simulink model "Three_blade_H_VAWT_Model"  (R2018b)
settings: Solver=FixedStepAuto  StartTime=0.0  StopTime=10  FixedStep=0.01  RelTol=1e-3
values from neighbouring files (symbols this model uses):
  A0 = 0    [Three_blade_H_VAWT_init.m]    (also in Three_blade_H_VAWT_pre_post.m)
  a1 = 0.01    [Three_blade_H_VAWT_init.m]    (also in Three_blade_H_VAWT_pre_post.m)
  a11 = 0.8    [Three_blade_H_VAWT_init.m]    (also in Three_blade_H_VAWT_pre_post.m)
  a12 = 0.2    [Three_blade_H_VAWT_init.m]    (also in Three_blade_H_VAWT_pre_post.m)
  a2 = 0.08    [Three_blade_H_VAWT_init.m]    (also in Three_blade_H_VAWT_pre_post.m)
  a21 = 0.5    [Three_blade_H_VAWT_init.m]    (also in Three_blade_H_VAWT_pre_post.m)
  a22 = 0.5    [Three_blade_H_VAWT_init.m]    (also in Three_blade_H_VAWT_pre_post.m)
  A_wind = 10    [Three_blade_H_VAWT_init.m]    (also in Three_blade_H_VAWT_pre_post.m)
  ACD1 = 12    [Three_blade_H_VAWT_init.m]    (also in Three_blade_H_VAWT_pre_post.m)
  ACL1 = 15    [Three_blade_H_VAWT_init.m]    (also in Three_blade_H_VAWT_pre_post.m)
  AR = Blade_Length/Chord    (= 10)    [Three_blade_H_VAWT_init.m]    (also in Three_blade_H_VAWT_pre_post.m = 40)
  blade1_pitch = 0    [Three_blade_H_VAWT_pre_post.m]
  blade1_radius = 20    [Three_blade_H_VAWT_pre_post.m]
  blade2_pitch = 0    [Three_blade_H_VAWT_pre_post.m]
  blade2_radius = 20    [Three_blade_H_VAWT_pre_post.m]
  blade3_pitch = 0    [Three_blade_H_VAWT_pre_post.m]
  blade3_radius = 20    [Three_blade_H_VAWT_pre_post.m]
  Blade_Length = 40    [Three_blade_H_VAWT_init.m]    (also in Three_blade_H_VAWT_pre_post.m)
  C_l_NACA0012_spline = spline(angles, C_l_NACA0012, [0:1:360])    [Three_blade_H_VAWT_init.m]    (also in Three_blade_H_VAWT_pre_post.m)
  CD0 = 0.005    [Three_blade_H_VAWT_init.m]    (also in Three_blade_H_VAWT_pre_post.m)
  CD1_max = 0.017    [Three_blade_H_VAWT_init.m]    (also in Three_blade_H_VAWT_pre_post.m)
  CD2_max = 1.8    [Three_blade_H_VAWT_init.m]    (also in Three_blade_H_VAWT_pre_post.m)
  CL1_max = 1.4    [Three_blade_H_VAWT_init.m]    (also in Three_blade_H_VAWT_pre_post.m)
  CL2_max = 1.2    [Three_blade_H_VAWT_init.m]    (also in Three_blade_H_VAWT_pre_post.m)
  D = 10^6    (= 1000000)    [Three_blade_H_VAWT_init.m]    (also in Three_blade_H_VAWT_pre_post.m)
  eta_g = 0.9    [Three_blade_H_VAWT_init.m]    (also in Three_blade_H_VAWT_pre_post.m)
  h1 = 1    [Three_blade_H_VAWT_init.m]    (also in Three_blade_H_VAWT_pre_post.m)
  h2 = 1    [Three_blade_H_VAWT_init.m]    (also in Three_blade_H_VAWT_pre_post.m)
  Jg = 15.8    [Three_blade_H_VAWT_init.m]    (also in Three_blade_H_VAWT_pre_post.m)
  K = 6*10^7    (= 60000000)    [Three_blade_H_VAWT_init.m]    (also in Three_blade_H_VAWT_pre_post.m)
  N = 100    [Three_blade_H_VAWT_init.m]    (also in Three_blade_H_VAWT_pre_post.m)
  phi11 = 0    [Three_blade_H_VAWT_init.m]    (also in Three_blade_H_VAWT_pre_post.m)
  phi12 = pi/2    (= 1.57079632679)    [Three_blade_H_VAWT_init.m]    (also in Three_blade_H_VAWT_pre_post.m)
  phi21 = 0    [Three_blade_H_VAWT_init.m]    (also in Three_blade_H_VAWT_pre_post.m)
  phi22 = pi/2    (= 1.57079632679)    [Three_blade_H_VAWT_init.m]    (also in Three_blade_H_VAWT_pre_post.m)
  Planform_A = Blade_Length*Chord    (= 160)    [Three_blade_H_VAWT_init.m]    (also in Three_blade_H_VAWT_pre_post.m = 40)
  rho = 1.225    [Three_blade_H_VAWT_init.m]    (also in Three_blade_H_VAWT_pre_post.m; sim_init_junior_project.m)
  S1 = 0.6/6    (= 0.1)    [Three_blade_H_VAWT_init.m]    (also in Three_blade_H_VAWT_pre_post.m)
  v_gustmax = v_wind    (= 5)    [Three_blade_H_VAWT_init.m]    (also in Three_blade_H_VAWT_pre_post.m)
  v_wind = 5    [Three_blade_H_VAWT_init.m]    (also in Three_blade_H_VAWT_pre_post.m)
  w_gust = (2*pi)/(30)    (= 0.209439510239)    [Three_blade_H_VAWT_init.m]    (also in Three_blade_H_VAWT_pre_post.m)
  w_wind = (2*pi)*5    (= 31.4159265359)    [Three_blade_H_VAWT_init.m]    (also in Three_blade_H_VAWT_pre_post.m)
  wind_vector_i = [50,0,0]    [Three_blade_H_VAWT_pre_post.m]
undefined symbols (not defined in the file or in its folder): Bg, C_Tg, C_Tr, c_wg, c_wr, Cg, Cr, J_g, Kg, Kr, L, magnitude, R2, Re, tau_e
libraries: vrlib x6, dspmathops x6
(part 2 of 2)

== system Three_blade_H_VAWT_Model/3bladeHVAWT with Generator/Blade Aerodymanics/Pre//Post Stall Foil Model NACA 0012/CD2 (post-stall) 1 ==
  alpha : Inport
  Abs : Abs
  CD2_max : Constant  Value=CD2_max
  Constant : Constant  Value=CD1_max
  Constant1 : Constant  Value=ACD1
  Constant2 : Constant  Value=90
  Constant3 : Constant  Value=ACD1
  Divide : Product  Inputs=**/
  Gain : Gain  Gain=pi/180
  MATLAB Function : MATLAB Function  TreatAsAtomicUnit=on
  Product : Product
  Product1 : Product
  Scope : Scope
  Sum : Sum  Inputs=|++
  Sum1 : Sum  Inputs=|+-
  Sum2 : Sum  Inputs=|+-
  Sum3 : Sum  Inputs=|+-
  Trigonometric Function : Trigonometry
  Cd : Outport
  wires:
  Constant/1 -> Sum/2, Sum1/2
  CD2_max/1 -> Sum1/1
  Sum1/1 -> Product/2
  Trigonometric Function/1 -> Product/1
  Product/1 -> Sum/1
  alpha/1 -> MATLAB Function/1(alpha), Sum2/1
  Constant1/1 -> Sum3/2, Sum2/2
  Constant2/1 -> Divide/2, Sum3/1
  Sum3/1 -> Divide/3
  Sum2/1 -> Divide/1
  Divide/1 -> Gain/1
  Gain/1 -> Trigonometric Function/1
  Product1/1 -> Abs/1
  Abs/1 -> Cd/1
  Constant3/1 -> MATLAB Function/2(ACD1)
  Sum/1 -> Product1/2
  MATLAB Function/1(y) -> Scope/1, Product1/1

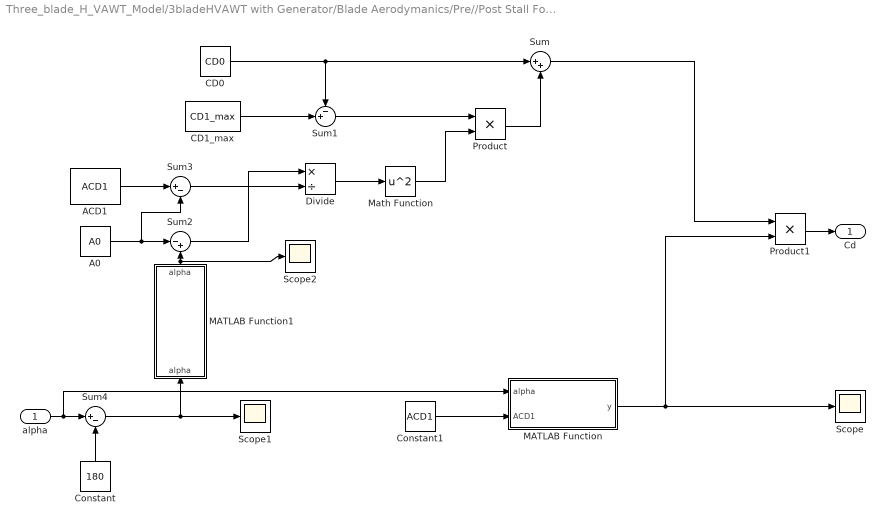
== system Three_blade_H_VAWT_Model/3bladeHVAWT with Generator/Blade Aerodymanics/Pre//Post Stall Foil Model NACA 0012/CD2 (post-stall) 2 ==
  alpha : Inport
  A0 : Constant  Value=A0
  ACD1 : Constant  Value=ACD1
  CD0 : Constant  Value=CD0
  CD1_max : Constant  Value=CD1_max
  Constant : Constant  Value=180
  Constant1 : Constant  Value=ACD1
  Divide : Product  Inputs=*/
  MATLAB Function : MATLAB Function  TreatAsAtomicUnit=on
  MATLAB Function1 : MATLAB Function  TreatAsAtomicUnit=on
  Math Function : Math  Operator=square  SaturateOnIntegerOverflow=on
  Product : Product
  Product1 : Product
  Scope : Scope
  Scope1 : Scope
  Scope2 : Scope
  Sum : Sum  Inputs=|++
  Sum1 : Sum  Inputs=-+|
  Sum2 : Sum  Inputs=|-+
  Sum3 : Sum  Inputs=|+-
  Sum4 : Sum  Inputs=|+-
  Cd : Outport
  wires:
  MATLAB Function1/1(alpha) -> Sum2/2, Scope2/1
  MATLAB Function/1(y) -> Scope/1, Product1/2
  Constant1/1 -> MATLAB Function/2(ACD1)
  Product1/1 -> Cd/1
  Sum/1 -> Product1/1
  Product/1 -> Sum/2
  Math Function/1 -> Product/2
  Divide/1 -> Math Function/1
  Sum3/1 -> Divide/2
  Sum2/1 -> Divide/1
  ACD1/1 -> Sum3/1
  A0/1 -> Sum2/1, Sum3/2
  Sum1/1 -> Product/1
  CD1_max/1 -> Sum1/2
  CD0/1 -> Sum/1, Sum1/1
  alpha/1 -> MATLAB Function/1(alpha), Sum4/1
  Sum4/1 -> Scope1/1, MATLAB Function1/1("alpha ")
  Constant/1 -> Sum4/2

== system Three_blade_H_VAWT_Model/3bladeHVAWT with Generator/Blade Aerodymanics/Pre//Post Stall Foil Model NACA 0012/CD2 (post-stall) 3 ==
  alpha : Inport
  Abs : Abs
  CD2_max : Constant  Value=CD2_max
  Constant : Constant  Value=CD1_max
  Constant1 : Constant  Value=ACD1
  Constant2 : Constant  Value=90
  Constant3 : Constant  Value=ACD1
  Constant4 : Constant  Value=-180
  Divide : Product  Inputs=**/
  Gain : Gain  Gain=pi/180
  MATLAB Function : MATLAB Function  TreatAsAtomicUnit=on
  Product : Product
  Product1 : Product
  Scope : Scope
  Sum : Sum  Inputs=|++
  Sum1 : Sum  Inputs=|+-
  Sum2 : Sum  Inputs=|+-
  Sum3 : Sum  Inputs=|+-
  Sum4 : Sum  Inputs=++|
  Trigonometric Function : Trigonometry
  Cd : Outport
  wires:
  MATLAB Function/1(y) -> Product1/1, Scope/1
  Sum/1 -> Product1/2
  Constant3/1 -> MATLAB Function/2(ACD1)
  Abs/1 -> Cd/1
  Product1/1 -> Abs/1
  Gain/1 -> Trigonometric Function/1
  Divide/1 -> Gain/1
  Sum2/1 -> Sum4/2
  Sum3/1 -> Divide/3
  Constant2/1 -> Sum3/1, Divide/2
  Constant1/1 -> Sum2/2, Sum3/2
  alpha/1 -> Sum2/1, MATLAB Function/1(alpha)
  Product/1 -> Sum/1
  Trigonometric Function/1 -> Product/1
  Sum1/1 -> Product/2
  CD2_max/1 -> Sum1/1
  Constant/1 -> Sum1/2, Sum/2
  Constant4/1 -> Sum4/1
  Sum4/1 -> Divide/1

== system Three_blade_H_VAWT_Model/3bladeHVAWT with Generator/Blade Aerodymanics/Pre//Post Stall Foil Model NACA 0012/CL1 (pre-stall) 1 ==
  alpha : Inport
  A0 : Constant  Value=A0
  A0 1 : Constant  Value=A0
  A0 2 : Constant  Value=A0
  ACl1 : Constant  Value=ACL1
  Cl1max : Constant  Value=CL1_max
  Constant : Constant
  Divide : Product  Inputs=/*
  Divide1 : Product  Inputs=*/
  Math Function : Math  Operator=pow  SaturateOnIntegerOverflow=on
  Product : Product
  Product1 : Product
  Product2 : Product
  S1 : Constant  Value=S1
  Sum{,1,3..4} (4 alike) : Sum  Inputs=|+-
  Sum2 : Sum  Inputs=|++
  Sum5 : Sum  Inputs=-+|
  Cl : Outport
  wires:
  alpha/1 -> Sum3/1
  ACl1/1 -> Sum/1, Sum4/1
  A0/1 -> Sum/2
  Cl1max/1 -> Sum1/2, Divide/2
  Sum/1 -> Product/2
  S1/1 -> Product/1, Product1/2
  Product/1 -> Sum1/1
  Sum1/1 -> Divide/1, Product2/2  "RCl1"
  Divide/1 -> Sum2/1
  Constant/1 -> Sum2/2
  Sum2/1 -> Math Function/2  "N1"
  A0 1/1 -> Sum3/2
  Sum3/1 -> Divide1/1, Product1/1
  Product1/1 -> Sum5/2
  Sum4/1 -> Divide1/2
  A0 2/1 -> Sum4/2
  Divide1/1 -> Math Function/1
  Math Function/1 -> Product2/1
  Product2/1 -> Sum5/1
  Sum5/1 -> Cl/1

== system Three_blade_H_VAWT_Model/3bladeHVAWT with Generator/Blade Aerodymanics/Pre//Post Stall Foil Model NACA 0012/CL2 (post-stall) 1 ==
  alpha : Inport
  Constant : Constant  Value=92
  Constant1 : Constant  Value=1.632
  Constant2 : Constant  Value=CL2_max
  Constant3 : Constant
  Divide : Product  Inputs=*/
  Gain : Gain  Gain=-0.032
  Gain1 : Gain  Gain=-1
  Gain2 : Gain  Gain=-1/51
  Math Function : Math  Operator=pow  SaturateOnIntegerOverflow=on
  Product : Product
  Sum : Sum  Inputs=|+-
  Sum1 : Sum  Inputs=|+-
  Sum2 : Sum  Inputs=|++
  Sum3 : Sum  Inputs=|++
  CL2 : Outport
  wires:
  alpha/1 -> Sum/1
  Constant/1 -> Sum/2
  Sum/1 -> Gain2/1, Gain/1
  Constant1/1 -> Sum1/1
  Constant2/1 -> Sum1/2, Divide/2
  Sum1/1 -> Gain1/1, Divide/1  "RCL2"
  Constant3/1 -> Sum2/1
  Divide/1 -> Sum2/2
  Sum2/1 -> Math Function/2  "N2"
  Gain1/1 -> Product/1
  Gain2/1 -> Math Function/1
  Math Function/1 -> Product/2
  Gain/1 -> Sum3/1
  Product/1 -> Sum3/2
  Sum3/1 -> CL2/1

== system Three_blade_H_VAWT_Model/3bladeHVAWT with Generator/Blade Aerodymanics/Pre//Post Stall Foil Model NACA 0012 (2)/CD1 (pre-stall) 1 ==
  alpha : Inport
  A0 : Constant  Value=A0
  ACD1 : Constant  Value=ACD1
  CD0 : Constant  Value=CD0
  CD1_max : Constant  Value=CD1_max
  Constant1 : Constant  Value=ACD1
  Divide : Product  Inputs=*/
  MATLAB Function : MATLAB Function  TreatAsAtomicUnit=on
  MATLAB Function1 : MATLAB Function  TreatAsAtomicUnit=on
  Math Function : Math  Operator=square  SaturateOnIntegerOverflow=on
  Product : Product
  Product1 : Product
  Scope : Scope
  Scope1 : Scope
  Scope2 : Scope
  Sum : Sum  Inputs=|++
  Sum1 : Sum  Inputs=-+|
  Sum2 : Sum  Inputs=|-+
  Sum3 : Sum  Inputs=|+-
  Cd : Outport
  wires:
  MATLAB Function1/1(alpha) -> Sum2/2, Scope2/1
  MATLAB Function/1(y) -> Scope/1, Product1/2
  Constant1/1 -> MATLAB Function/2(ACD1)
  Product1/1 -> Cd/1
  Sum/1 -> Product1/1
  Product/1 -> Sum/2
  Math Function/1 -> Product/2
  Divide/1 -> Math Function/1
  Sum3/1 -> Divide/2
  Sum2/1 -> Divide/1
  ACD1/1 -> Sum3/1
  A0/1 -> Sum2/1, Sum3/2
  Sum1/1 -> Product/1
  CD1_max/1 -> Sum1/2
  CD0/1 -> Sum/1, Sum1/1
  alpha/1 -> MATLAB Function1/1("alpha "), Scope1/1, MATLAB Function/1(alpha)

== system Three_blade_H_VAWT_Model/3bladeHVAWT with Generator/Blade Aerodymanics/Pre//Post Stall Foil Model NACA 0012 (2)/CD2 (post-stall) 1 ==
  alpha : Inport
  Abs : Abs
  CD2_max : Constant  Value=CD2_max
  Constant : Constant  Value=CD1_max
  Constant1 : Constant  Value=ACD1
  Constant2 : Constant  Value=90
  Constant3 : Constant  Value=ACD1
  Divide : Product  Inputs=**/
  Gain : Gain  Gain=pi/180
  MATLAB Function : MATLAB Function  TreatAsAtomicUnit=on
  Product : Product
  Product1 : Product
  Scope : Scope
  Sum : Sum  Inputs=|++
  Sum1 : Sum  Inputs=|+-
  Sum2 : Sum  Inputs=|+-
  Sum3 : Sum  Inputs=|+-
  Trigonometric Function : Trigonometry
  Cd : Outport
  wires:
  MATLAB Function/1(y) -> Product1/1, Scope/1
  Sum/1 -> Product1/2
  Constant3/1 -> MATLAB Function/2(ACD1)
  Abs/1 -> Cd/1
  Product1/1 -> Abs/1
  Gain/1 -> Trigonometric Function/1
  Divide/1 -> Gain/1
  Sum2/1 -> Divide/1
  Sum3/1 -> Divide/3
  Constant2/1 -> Sum3/1, Divide/2
  Constant1/1 -> Sum2/2, Sum3/2
  alpha/1 -> Sum2/1, MATLAB Function/1(alpha)
  Product/1 -> Sum/1
  Trigonometric Function/1 -> Product/1
  Sum1/1 -> Product/2
  CD2_max/1 -> Sum1/1
  Constant/1 -> Sum1/2, Sum/2

== system Three_blade_H_VAWT_Model/3bladeHVAWT with Generator/Blade Aerodymanics/Pre//Post Stall Foil Model NACA 0012 (2)/CD2 (post-stall) 2 ==
  alpha : Inport
  A0 : Constant  Value=A0
  ACD1 : Constant  Value=ACD1
  CD0 : Constant  Value=CD0
  CD1_max : Constant  Value=CD1_max
  Constant : Constant  Value=180
  Constant1 : Constant  Value=ACD1
  Divide : Product  Inputs=*/
  MATLAB Function : MATLAB Function  TreatAsAtomicUnit=on
  MATLAB Function1 : MATLAB Function  TreatAsAtomicUnit=on
  Math Function : Math  Operator=square  SaturateOnIntegerOverflow=on
  Product : Product
  Product1 : Product
  Scope : Scope
  Scope1 : Scope
  Scope2 : Scope
  Sum : Sum  Inputs=|++
  Sum1 : Sum  Inputs=-+|
  Sum2 : Sum  Inputs=|-+
  Sum3 : Sum  Inputs=|+-
  Sum4 : Sum  Inputs=|+-
  Cd : Outport
  wires:
  Constant/1 -> Sum4/2
  Sum4/1 -> MATLAB Function1/1("alpha "), Scope1/1
  alpha/1 -> Sum4/1, MATLAB Function/1(alpha)
  CD0/1 -> Sum1/1, Sum/1
  CD1_max/1 -> Sum1/2
  Sum1/1 -> Product/1
  A0/1 -> Sum3/2, Sum2/1
  ACD1/1 -> Sum3/1
  Sum2/1 -> Divide/1
  Sum3/1 -> Divide/2
  Divide/1 -> Math Function/1
  Math Function/1 -> Product/2
  Product/1 -> Sum/2
  Sum/1 -> Product1/1
  Product1/1 -> Cd/1
  Constant1/1 -> MATLAB Function/2(ACD1)
  MATLAB Function/1(y) -> Product1/2, Scope/1
  MATLAB Function1/1(alpha) -> Scope2/1, Sum2/2

== system Three_blade_H_VAWT_Model/3bladeHVAWT with Generator/Blade Aerodymanics/Pre//Post Stall Foil Model NACA 0012 (2)/CD2 (post-stall) 3 ==
  alpha : Inport
  Abs : Abs
  CD2_max : Constant  Value=CD2_max
  Constant : Constant  Value=CD1_max
  Constant1 : Constant  Value=ACD1
  Constant2 : Constant  Value=90
  Constant3 : Constant  Value=ACD1
  Constant4 : Constant  Value=-180
  Divide : Product  Inputs=**/
  Gain : Gain  Gain=pi/180
  MATLAB Function : MATLAB Function  TreatAsAtomicUnit=on
  Product : Product
  Product1 : Product
  Scope : Scope
  Sum : Sum  Inputs=|++
  Sum1 : Sum  Inputs=|+-
  Sum2 : Sum  Inputs=|+-
  Sum3 : Sum  Inputs=|+-
  Sum4 : Sum  Inputs=++|
  Trigonometric Function : Trigonometry
  Cd : Outport
  wires:
  Sum4/1 -> Divide/1
  Constant4/1 -> Sum4/1
  Constant/1 -> Sum/2, Sum1/2
  CD2_max/1 -> Sum1/1
  Sum1/1 -> Product/2
  Trigonometric Function/1 -> Product/1
  Product/1 -> Sum/1
  alpha/1 -> MATLAB Function/1(alpha), Sum2/1
  Constant1/1 -> Sum3/2, Sum2/2
  Constant2/1 -> Divide/2, Sum3/1
  Sum3/1 -> Divide/3
  Sum2/1 -> Sum4/2
  Divide/1 -> Gain/1
  Gain/1 -> Trigonometric Function/1
  Product1/1 -> Abs/1
  Abs/1 -> Cd/1
  Constant3/1 -> MATLAB Function/2(ACD1)
  Sum/1 -> Product1/2
  MATLAB Function/1(y) -> Scope/1, Product1/1

== system Three_blade_H_VAWT_Model/3bladeHVAWT with Generator/Blade Aerodymanics/Pre//Post Stall Foil Model NACA 0012 (2)/CL1 (pre-stall) 1 ==
  alpha : Inport
  A0 : Constant  Value=A0
  A0 1 : Constant  Value=A0
  A0 2 : Constant  Value=A0
  ACl1 : Constant  Value=ACL1
  Cl1max : Constant  Value=CL1_max
  Constant : Constant
  Divide : Product  Inputs=/*
  Divide1 : Product  Inputs=*/
  Math Function : Math  Operator=pow  SaturateOnIntegerOverflow=on
  Product : Product
  Product1 : Product
  Product2 : Product
  S1 : Constant  Value=S1
  Sum{,1,3..4} (4 alike) : Sum  Inputs=|+-
  Sum2 : Sum  Inputs=|++
  Sum5 : Sum  Inputs=-+|
  Cl : Outport
  wires:
  Sum5/1 -> Cl/1
  Product2/1 -> Sum5/1
  Math Function/1 -> Product2/1
  Divide1/1 -> Math Function/1
  A0 2/1 -> Sum4/2
  Sum4/1 -> Divide1/2
  Product1/1 -> Sum5/2
  Sum3/1 -> Product1/1, Divide1/1
  A0 1/1 -> Sum3/2
  Sum2/1 -> Math Function/2  "N1"
  Constant/1 -> Sum2/2
  Divide/1 -> Sum2/1
  Sum1/1 -> Product2/2, Divide/1  "RCl1"
  Product/1 -> Sum1/1
  S1/1 -> Product1/2, Product/1
  Sum/1 -> Product/2
  Cl1max/1 -> Divide/2, Sum1/2
  A0/1 -> Sum/2
  ACl1/1 -> Sum4/1, Sum/1
  alpha/1 -> Sum3/1

== system Three_blade_H_VAWT_Model/3bladeHVAWT with Generator/Blade Aerodymanics/Pre//Post Stall Foil Model NACA 0012 (2)/CL2 (post-stall) 1 ==
  alpha : Inport
  Constant : Constant  Value=92
  Constant1 : Constant  Value=1.632
  Constant2 : Constant  Value=CL2_max
  Constant3 : Constant
  Divide : Product  Inputs=*/
  Gain : Gain  Gain=-0.032
  Gain1 : Gain  Gain=-1
  Gain2 : Gain  Gain=-1/51
  Math Function : Math  Operator=pow  SaturateOnIntegerOverflow=on
  Product : Product
  Sum : Sum  Inputs=|+-
  Sum1 : Sum  Inputs=|+-
  Sum2 : Sum  Inputs=|++
  Sum3 : Sum  Inputs=|++
  CL2 : Outport
  wires:
  Sum3/1 -> CL2/1
  Product/1 -> Sum3/2
  Gain/1 -> Sum3/1
  Math Function/1 -> Product/2
  Gain2/1 -> Math Function/1
  Gain1/1 -> Product/1
  Sum2/1 -> Math Function/2  "N2"
  Divide/1 -> Sum2/2
  Constant3/1 -> Sum2/1
  Sum1/1 -> Divide/1, Gain1/1  "RCL2"
  Constant2/1 -> Divide/2, Sum1/2
  Constant1/1 -> Sum1/1
  Sum/1 -> Gain/1, Gain2/1
  Constant/1 -> Sum/2
  alpha/1 -> Sum/1

== system Three_blade_H_VAWT_Model/3bladeHVAWT with Generator/Blade Aerodymanics/Pre//Post Stall Foil Model NACA 0012 (3)/CD1 (pre-stall) 1 ==
  alpha : Inport
  A0 : Constant  Value=A0
  ACD1 : Constant  Value=ACD1
  CD0 : Constant  Value=CD0
  CD1_max : Constant  Value=CD1_max
  Constant1 : Constant  Value=ACD1
  Divide : Product  Inputs=*/
  MATLAB Function : MATLAB Function  TreatAsAtomicUnit=on
  MATLAB Function1 : MATLAB Function  TreatAsAtomicUnit=on
  Math Function : Math  Operator=square  SaturateOnIntegerOverflow=on
  Product : Product
  Product1 : Product
  Scope : Scope
  Scope1 : Scope
  Scope2 : Scope
  Sum : Sum  Inputs=|++
  Sum1 : Sum  Inputs=-+|
  Sum2 : Sum  Inputs=|-+
  Sum3 : Sum  Inputs=|+-
  Cd : Outport
  wires:
  alpha/1 -> MATLAB Function/1(alpha), Scope1/1, MATLAB Function1/1("alpha ")
  CD0/1 -> Sum1/1, Sum/1
  CD1_max/1 -> Sum1/2
  Sum1/1 -> Product/1
  A0/1 -> Sum3/2, Sum2/1
  ACD1/1 -> Sum3/1
  Sum2/1 -> Divide/1
  Sum3/1 -> Divide/2
  Divide/1 -> Math Function/1
  Math Function/1 -> Product/2
  Product/1 -> Sum/2
  Sum/1 -> Product1/1
  Product1/1 -> Cd/1
  Constant1/1 -> MATLAB Function/2(ACD1)
  MATLAB Function/1(y) -> Product1/2, Scope/1
  MATLAB Function1/1(alpha) -> Scope2/1, Sum2/2

== system Three_blade_H_VAWT_Model/3bladeHVAWT with Generator/Blade Aerodymanics/Pre//Post Stall Foil Model NACA 0012 (3)/CD2 (post-stall) 1 ==
  alpha : Inport
  Abs : Abs
  CD2_max : Constant  Value=CD2_max
  Constant : Constant  Value=CD1_max
  Constant1 : Constant  Value=ACD1
  Constant2 : Constant  Value=90
  Constant3 : Constant  Value=ACD1
  Divide : Product  Inputs=**/
  Gain : Gain  Gain=pi/180
  MATLAB Function : MATLAB Function  TreatAsAtomicUnit=on
  Product : Product
  Product1 : Product
  Scope : Scope
  Sum : Sum  Inputs=|++
  Sum1 : Sum  Inputs=|+-
  Sum2 : Sum  Inputs=|+-
  Sum3 : Sum  Inputs=|+-
  Trigonometric Function : Trigonometry
  Cd : Outport
  wires:
  Constant/1 -> Sum/2, Sum1/2
  CD2_max/1 -> Sum1/1
  Sum1/1 -> Product/2
  Trigonometric Function/1 -> Product/1
  Product/1 -> Sum/1
  alpha/1 -> MATLAB Function/1(alpha), Sum2/1
  Constant1/1 -> Sum3/2, Sum2/2
  Constant2/1 -> Divide/2, Sum3/1
  Sum3/1 -> Divide/3
  Sum2/1 -> Divide/1
  Divide/1 -> Gain/1
  Gain/1 -> Trigonometric Function/1
  Product1/1 -> Abs/1
  Abs/1 -> Cd/1
  Constant3/1 -> MATLAB Function/2(ACD1)
  Sum/1 -> Product1/2
  MATLAB Function/1(y) -> Scope/1, Product1/1

== system Three_blade_H_VAWT_Model/3bladeHVAWT with Generator/Blade Aerodymanics/Pre//Post Stall Foil Model NACA 0012 (3)/CD2 (post-stall) 2 ==
  alpha : Inport
  A0 : Constant  Value=A0
  ACD1 : Constant  Value=ACD1
  CD0 : Constant  Value=CD0
  CD1_max : Constant  Value=CD1_max
  Constant : Constant  Value=180
  Constant1 : Constant  Value=ACD1
  Divide : Product  Inputs=*/
  MATLAB Function : MATLAB Function  TreatAsAtomicUnit=on
  MATLAB Function1 : MATLAB Function  TreatAsAtomicUnit=on
  Math Function : Math  Operator=square  SaturateOnIntegerOverflow=on
  Product : Product
  Product1 : Product
  Scope : Scope
  Scope1 : Scope
  Scope2 : Scope
  Sum : Sum  Inputs=|++
  Sum1 : Sum  Inputs=-+|
  Sum2 : Sum  Inputs=|-+
  Sum3 : Sum  Inputs=|+-
  Sum4 : Sum  Inputs=|+-
  Cd : Outport
  wires:
  MATLAB Function1/1(alpha) -> Sum2/2, Scope2/1
  MATLAB Function/1(y) -> Scope/1, Product1/2
  Constant1/1 -> MATLAB Function/2(ACD1)
  Product1/1 -> Cd/1
  Sum/1 -> Product1/1
  Product/1 -> Sum/2
  Math Function/1 -> Product/2
  Divide/1 -> Math Function/1
  Sum3/1 -> Divide/2
  Sum2/1 -> Divide/1
  ACD1/1 -> Sum3/1
  A0/1 -> Sum2/1, Sum3/2
  Sum1/1 -> Product/1
  CD1_max/1 -> Sum1/2
  CD0/1 -> Sum/1, Sum1/1
  alpha/1 -> MATLAB Function/1(alpha), Sum4/1
  Sum4/1 -> Scope1/1, MATLAB Function1/1("alpha ")
  Constant/1 -> Sum4/2

== system Three_blade_H_VAWT_Model/3bladeHVAWT with Generator/Blade Aerodymanics/Pre//Post Stall Foil Model NACA 0012 (3)/CD2 (post-stall) 3 ==
  alpha : Inport
  Abs : Abs
  CD2_max : Constant  Value=CD2_max
  Constant : Constant  Value=CD1_max
  Constant1 : Constant  Value=ACD1
  Constant2 : Constant  Value=90
  Constant3 : Constant  Value=ACD1
  Constant4 : Constant  Value=-180
  Divide : Product  Inputs=**/
  Gain : Gain  Gain=pi/180
  MATLAB Function : MATLAB Function  TreatAsAtomicUnit=on
  Product : Product
  Product1 : Product
  Scope : Scope
  Sum : Sum  Inputs=|++
  Sum1 : Sum  Inputs=|+-
  Sum2 : Sum  Inputs=|+-
  Sum3 : Sum  Inputs=|+-
  Sum4 : Sum  Inputs=++|
  Trigonometric Function : Trigonometry
  Cd : Outport
  wires:
  MATLAB Function/1(y) -> Product1/1, Scope/1
  Sum/1 -> Product1/2
  Constant3/1 -> MATLAB Function/2(ACD1)
  Abs/1 -> Cd/1
  Product1/1 -> Abs/1
  Gain/1 -> Trigonometric Function/1
  Divide/1 -> Gain/1
  Sum2/1 -> Sum4/2
  Sum3/1 -> Divide/3
  Constant2/1 -> Sum3/1, Divide/2
  Constant1/1 -> Sum2/2, Sum3/2
  alpha/1 -> Sum2/1, MATLAB Function/1(alpha)
  Product/1 -> Sum/1
  Trigonometric Function/1 -> Product/1
  Sum1/1 -> Product/2
  CD2_max/1 -> Sum1/1
  Constant/1 -> Sum1/2, Sum/2
  Constant4/1 -> Sum4/1
  Sum4/1 -> Divide/1

== system Three_blade_H_VAWT_Model/3bladeHVAWT with Generator/Blade Aerodymanics/Pre//Post Stall Foil Model NACA 0012 (3)/CL1 (pre-stall) 1 ==
  alpha : Inport
  A0 : Constant  Value=A0
  A0 1 : Constant  Value=A0
  A0 2 : Constant  Value=A0
  ACl1 : Constant  Value=ACL1
  Cl1max : Constant  Value=CL1_max
  Constant : Constant
  Divide : Product  Inputs=/*
  Divide1 : Product  Inputs=*/
  Math Function : Math  Operator=pow  SaturateOnIntegerOverflow=on
  Product : Product
  Product1 : Product
  Product2 : Product
  S1 : Constant  Value=S1
  Sum{,1,3..4} (4 alike) : Sum  Inputs=|+-
  Sum2 : Sum  Inputs=|++
  Sum5 : Sum  Inputs=-+|
  Cl : Outport
  wires:
  alpha/1 -> Sum3/1
  ACl1/1 -> Sum/1, Sum4/1
  A0/1 -> Sum/2
  Cl1max/1 -> Sum1/2, Divide/2
  Sum/1 -> Product/2
  S1/1 -> Product/1, Product1/2
  Product/1 -> Sum1/1
  Sum1/1 -> Divide/1, Product2/2  "RCl1"
  Divide/1 -> Sum2/1
  Constant/1 -> Sum2/2
  Sum2/1 -> Math Function/2  "N1"
  A0 1/1 -> Sum3/2
  Sum3/1 -> Divide1/1, Product1/1
  Product1/1 -> Sum5/2
  Sum4/1 -> Divide1/2
  A0 2/1 -> Sum4/2
  Divide1/1 -> Math Function/1
  Math Function/1 -> Product2/1
  Product2/1 -> Sum5/1
  Sum5/1 -> Cl/1

== system Three_blade_H_VAWT_Model/3bladeHVAWT with Generator/Blade Aerodymanics/Pre//Post Stall Foil Model NACA 0012 (3)/CL2 (post-stall) 1 ==
  alpha : Inport
  Constant : Constant  Value=92
  Constant1 : Constant  Value=1.632
  Constant2 : Constant  Value=CL2_max
  Constant3 : Constant
  Divide : Product  Inputs=*/
  Gain : Gain  Gain=-0.032
  Gain1 : Gain  Gain=-1
  Gain2 : Gain  Gain=-1/51
  Math Function : Math  Operator=pow  SaturateOnIntegerOverflow=on
  Product : Product
  Sum : Sum  Inputs=|+-
  Sum1 : Sum  Inputs=|+-
  Sum2 : Sum  Inputs=|++
  Sum3 : Sum  Inputs=|++
  CL2 : Outport
  wires:
  alpha/1 -> Sum/1
  Constant/1 -> Sum/2
  Sum/1 -> Gain2/1, Gain/1
  Constant1/1 -> Sum1/1
  Constant2/1 -> Sum1/2, Divide/2
  Sum1/1 -> Gain1/1, Divide/1  "RCL2"
  Constant3/1 -> Sum2/1
  Divide/1 -> Sum2/2
  Sum2/1 -> Math Function/2  "N2"
  Gain1/1 -> Product/1
  Gain2/1 -> Math Function/1
  Math Function/1 -> Product/2
  Gain/1 -> Sum3/1
  Product/1 -> Sum3/2
  Sum3/1 -> CL2/1

== matlab function Three_blade_H_VAWT_Model/3bladeHVAWT with Generator/Blade Aerodymanics/Pre//Post Stall Foil Model NACA 0012/CD1 (pre-stall) 1/MATLAB Function1 ==
  data: alpha input; alpha output
function alpha   = fcn(alpha)

if alpha < 180
    alpha = alpha;
    
elseif alpha > 180
    alpha = -360 + alpha;
    
end

== matlab function Three_blade_H_VAWT_Model/3bladeHVAWT with Generator/Blade Aerodymanics/Pre//Post Stall Foil Model NACA 0012/CD1 (pre-stall) 1/MATLAB Function ==
  data: alpha input; y output; ACD1 input
function y = bandpass(alpha, ACD1)

if (ACD1-alpha) >= 0
    y = 1;
elseif (360-ACD1)-alpha <= 0
    y = 1;
else
    y = 0;
end
end

== matlab function Three_blade_H_VAWT_Model/3bladeHVAWT with Generator/Blade Aerodymanics/Pre//Post Stall Foil Model NACA 0012/CD2 (post-stall) 1/MATLAB Function ==
  data: alpha input; y output; ACD1 input
function y = bandpass(alpha, ACD1)

if (ACD1-alpha) >= 0
    y = 0;
elseif (180-ACD1)-alpha >=0
    y = 1;
elseif (ACD1+180-alpha) >=0
    y = 0;
elseif (360-ACD1-alpha) >=0
    y = 0;
else
    y = 0;
    
end

== matlab function Three_blade_H_VAWT_Model/3bladeHVAWT with Generator/Blade Aerodymanics/Pre//Post Stall Foil Model NACA 0012/CD2 (post-stall) 2/MATLAB Function ==
  data: alpha input; y output; ACD1 input
function y = bandpass(alpha, ACD1)

if (180-ACD1-alpha) >= 0
    y = 0;
elseif (180+ACD1)-alpha >= 0
    y = 1;
else
    y = 0;
end

== matlab function Three_blade_H_VAWT_Model/3bladeHVAWT with Generator/Blade Aerodymanics/Pre//Post Stall Foil Model NACA 0012/CD2 (post-stall) 2/MATLAB Function1 ==
  data: alpha input; alpha output
function alpha   = fcn(alpha)

if alpha < 180
    alpha = alpha;
    
elseif alpha > 180
    alpha = -360 + alpha;
    
end

== matlab function Three_blade_H_VAWT_Model/3bladeHVAWT with Generator/Blade Aerodymanics/Pre//Post Stall Foil Model NACA 0012/CD2 (post-stall) 3/MATLAB Function ==
  data: alpha input; y output; ACD1 input
function y = bandpass(alpha, ACD1)

if (ACD1-alpha) >= 0
    y = 0;
elseif (180-ACD1)-alpha >=0
    y = 0;
elseif (ACD1+180-alpha) >=0
    y = 0;
elseif (360-ACD1-alpha) >=0
    y = 1;
else
    y = 0;
    
end

== matlab function Three_blade_H_VAWT_Model/3bladeHVAWT with Generator/Blade Aerodymanics/Pre//Post Stall Foil Model NACA 0012 (2)/CD1 (pre-stall) 1/MATLAB Function ==
  data: alpha input; y output; ACD1 input
function y = bandpass(alpha, ACD1)

if (ACD1-alpha) >= 0
    y = 1;
elseif (360-ACD1)-alpha <= 0
    y = 1;
else
    y = 0;
end
end

== matlab function Three_blade_H_VAWT_Model/3bladeHVAWT with Generator/Blade Aerodymanics/Pre//Post Stall Foil Model NACA 0012 (2)/CD1 (pre-stall) 1/MATLAB Function1 ==
  data: alpha input; alpha output
function alpha   = fcn(alpha)

if alpha < 180
    alpha = alpha;
    
elseif alpha > 180
    alpha = -360 + alpha;
    
end

== matlab function Three_blade_H_VAWT_Model/3bladeHVAWT with Generator/Blade Aerodymanics/Pre//Post Stall Foil Model NACA 0012 (2)/CD2 (post-stall) 1/MATLAB Function ==
  data: alpha input; y output; ACD1 input
function y = bandpass(alpha, ACD1)

if (ACD1-alpha) >= 0
    y = 0;
elseif (180-ACD1)-alpha >=0
    y = 1;
elseif (ACD1+180-alpha) >=0
    y = 0;
elseif (360-ACD1-alpha) >=0
    y = 0;
else
    y = 0;
    
end

== matlab function Three_blade_H_VAWT_Model/3bladeHVAWT with Generator/Blade Aerodymanics/Pre//Post Stall Foil Model NACA 0012 (2)/CD2 (post-stall) 2/MATLAB Function ==
  data: alpha input; y output; ACD1 input
function y = bandpass(alpha, ACD1)

if (180-ACD1-alpha) >= 0
    y = 0;
elseif (180+ACD1)-alpha >= 0
    y = 1;
else
    y = 0;
end

== matlab function Three_blade_H_VAWT_Model/3bladeHVAWT with Generator/Blade Aerodymanics/Pre//Post Stall Foil Model NACA 0012 (2)/CD2 (post-stall) 2/MATLAB Function1 ==
  data: alpha input; alpha output
function alpha   = fcn(alpha)

if alpha < 180
    alpha = alpha;
    
elseif alpha > 180
    alpha = -360 + alpha;
    
end

== matlab function Three_blade_H_VAWT_Model/3bladeHVAWT with Generator/Blade Aerodymanics/Pre//Post Stall Foil Model NACA 0012 (2)/CD2 (post-stall) 3/MATLAB Function ==
  data: alpha input; y output; ACD1 input
function y = bandpass(alpha, ACD1)

if (ACD1-alpha) >= 0
    y = 0;
elseif (180-ACD1)-alpha >=0
    y = 0;
elseif (ACD1+180-alpha) >=0
    y = 0;
elseif (360-ACD1-alpha) >=0
    y = 1;
else
    y = 0;
    
end

== matlab function Three_blade_H_VAWT_Model/3bladeHVAWT with Generator/Blade Aerodymanics/Pre//Post Stall Foil Model NACA 0012 (3)/CD1 (pre-stall) 1/MATLAB Function ==
  data: alpha input; y output; ACD1 input
function y = bandpass(alpha, ACD1)

if (ACD1-alpha) >= 0
    y = 1;
elseif (360-ACD1)-alpha <= 0
    y = 1;
else
    y = 0;
end
end

== matlab function Three_blade_H_VAWT_Model/3bladeHVAWT with Generator/Blade Aerodymanics/Pre//Post Stall Foil Model NACA 0012 (3)/CD1 (pre-stall) 1/MATLAB Function1 ==
  data: alpha input; alpha output
function alpha   = fcn(alpha)

if alpha < 180
    alpha = alpha;
    
elseif alpha > 180
    alpha = -360 + alpha;
    
end

== matlab function Three_blade_H_VAWT_Model/3bladeHVAWT with Generator/Blade Aerodymanics/Pre//Post Stall Foil Model NACA 0012 (3)/CD2 (post-stall) 1/MATLAB Function ==
  data: alpha input; y output; ACD1 input
function y = bandpass(alpha, ACD1)

if (ACD1-alpha) >= 0
    y = 0;
elseif (180-ACD1)-alpha >=0
    y = 1;
elseif (ACD1+180-alpha) >=0
    y = 0;
elseif (360-ACD1-alpha) >=0
    y = 0;
else
    y = 0;
    
end

== matlab function Three_blade_H_VAWT_Model/3bladeHVAWT with Generator/Blade Aerodymanics/Pre//Post Stall Foil Model NACA 0012 (3)/CD2 (post-stall) 2/MATLAB Function ==
  data: alpha input; y output; ACD1 input
function y = bandpass(alpha, ACD1)

if (180-ACD1-alpha) >= 0
    y = 0;
elseif (180+ACD1)-alpha >= 0
    y = 1;
else
    y = 0;
end

== matlab function Three_blade_H_VAWT_Model/3bladeHVAWT with Generator/Blade Aerodymanics/Pre//Post Stall Foil Model NACA 0012 (3)/CD2 (post-stall) 2/MATLAB Function1 ==
  data: alpha input; alpha output
function alpha   = fcn(alpha)

if alpha < 180
    alpha = alpha;
    
elseif alpha > 180
    alpha = -360 + alpha;
    
end

== matlab function Three_blade_H_VAWT_Model/3bladeHVAWT with Generator/Blade Aerodymanics/Pre//Post Stall Foil Model NACA 0012 (3)/CD2 (post-stall) 3/MATLAB Function ==
  data: alpha input; y output; ACD1 input
function y = bandpass(alpha, ACD1)

if (ACD1-alpha) >= 0
    y = 0;
elseif (180-ACD1)-alpha >=0
    y = 0;
elseif (ACD1+180-alpha) >=0
    y = 0;
elseif (360-ACD1-alpha) >=0
    y = 1;
else
    y = 0;
    
end

== matlab function Three_blade_H_VAWT_Model/3bladeHVAWT with Generator/Blade Aerodymanics/Lift Align3/MATLAB Function ==
  data: Theta input; Mat output
function Mat = RotationMatrix(Theta)

Mat = [cos(Theta), -sin(Theta); sin(Theta), cos(Theta)];

== matlab function Three_blade_H_VAWT_Model/3bladeHVAWT with Generator/Blade Aerodymanics/Lift Align1/MATLAB Function ==
  data: Theta input; Mat output
function Mat = RotationMatrix(Theta)

Mat = [cos(Theta), -sin(Theta); sin(Theta), cos(Theta)];

== matlab function Three_blade_H_VAWT_Model/3bladeHVAWT with Generator/Blade Aerodymanics/Lift Align2/MATLAB Function ==
  data: Theta input; Mat output
function Mat = RotationMatrix(Theta)

Mat = [cos(Theta), -sin(Theta); sin(Theta), cos(Theta)];

== matlab function Three_blade_H_VAWT_Model/3bladeHVAWT with Generator/Blade Geometry Mk2/MATLAB Function ==
  data: Theta input; Mat output
function Mat = RotationMatrix(Theta)

Mat = [cos(Theta), -sin(Theta), 0
       sin(Theta), cos(Theta),  0
       0,          0,           1];
